simulink model "test"  (R2014a)
settings: Solver=ode3  StartTime=0.0  StopTime=100  RelTol=1e-3
libraries: slident x2, simulink x1
settings Model: Creator=admin  LastModifiedBy=admin

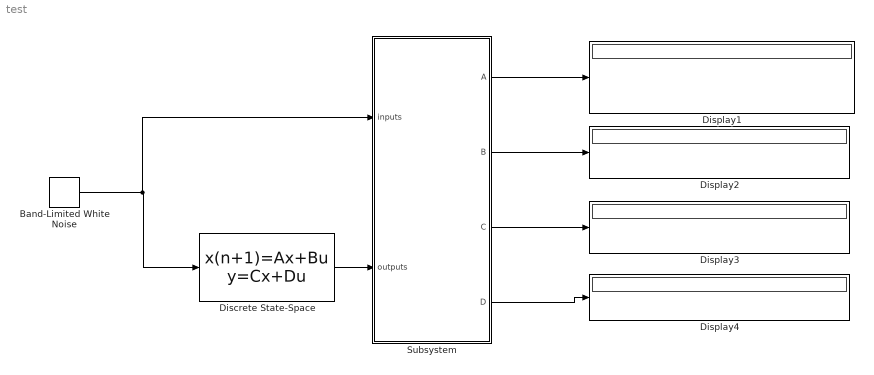
== system test ==
  Band-Limited White Noise : simulink/Sources/Band-Limited White Noise  Cov=[10]  Ts=1  seed=randi(10000)
  Discrete State-Space : DiscreteStateSpace  A=[11 1 0; 12 0 1; 13 0 0]  B=[1; 2; 3]  C=[1 0 0]  D=0
  Display{1..4} (4 alike) : Display
  Subsystem : Subsystem
  wires:
  Band-Limited White Noise/1 -> Discrete State-Space/1, Subsystem/1(inputs)
  Discrete State-Space/1 -> Subsystem/2(outputs)
  Subsystem/1(A) -> Display1/1
  Subsystem/2(B) -> Display2/1
  Subsystem/3(C) -> Display3/1
  Subsystem/4(D) -> Display4/1

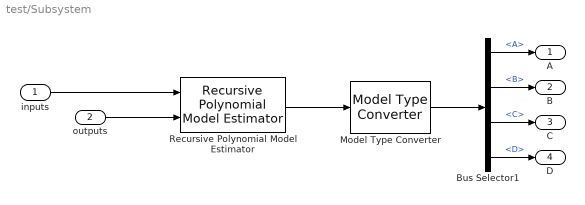
== system test/Subsystem ==
  inputs : Inport
  outputs : Inport  Port=2
  Bus Selector1 : BusSelector  OutputSignals=A,B,C,D
  Model Type Converter : slident/Estimators/Model Type Converter
  Recursive Polynomial Model Estimator : slident/Estimators/Recursive Polynomial Model Estimator  ModelStructure=ARMAX  InitialEstimateSource=None  A0=3  B0=1  C0=1  nk=3  P0=1e4  EstimationMethod=Forgetting Factor  AdaptationParameter=1  OutputError=off  OutputP=off  AddEnablePort=off  Ts=1
  A : Outport
  B : Outport  Port=2
  C : Outport  Port=3
  D : Outport  Port=4
  wires:
  Recursive Polynomial Model Estimator/1 -> Model Type Converter/1
  outputs/1 -> Recursive Polynomial Model Estimator/2
  inputs/1 -> Recursive Polynomial Model Estimator/1
  Model Type Converter/1 -> Bus Selector1/1
  Bus Selector1/1 -> A/1  "<A>"
  Bus Selector1/2 -> B/1  "<B>"
  Bus Selector1/3 -> C/1  "<C>"
  Bus Selector1/4 -> D/1  "<D>"
